simulink model "thrust_allocation"  (R2019a)
settings: Solver=FixedStepAuto  StartTime=0.0  StopTime=10.0  FixedStep=0.1  RelTol=1e-3
undefined symbols (not defined in the file or in its folder): thrusters
settings Model: Creator=den  LastModifiedBy=den

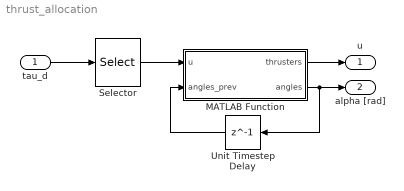
== system thrust_allocation ==
  tau_d : Inport
  MATLAB Function : MATLAB Function  TreatAsAtomicUnit=on
  Selector : Selector  InputPortWidth=6  IndexOptions=Index vector (dialog)  Indices=[1 2 6]  OutputSizes=1
  Unit Timestep Delay : Delay  DelayLength=1  InitialCondition=[thrusters.initangle]
  u : Outport
  alpha [rad] : Outport  Port=2
  wires:
  MATLAB Function/1(thrusters) -> u/1
  Selector/1 -> MATLAB Function/1(u)
  Unit Timestep Delay/1 -> MATLAB Function/2(angles_prev)
  tau_d/1 -> Selector/1
  MATLAB Function/2(angles) -> Unit Timestep Delay/1, alpha [rad]/1

== matlab function thrust_allocation/MATLAB Function ==
  data: u input; thrusters output; angles output; angles_prev input
function [thrusters, angles] = fcn(u, angles_prev)

% thrusters = load('thrusters_sup.mat');
% thrustLimits = [thrusters.thrust];
% throttleLimits = [thrusters.rate];
% turnLimit = [thrusters.rotationspeed];
% 
% % thruster positions
% tp = [thrusters.xposition; thrusters.yposition];

thrustLimits = [125000; 125000; 150000; 320000; 320000];
throttleLimits = [15625; 15625; 18750; 32000; 32000];
turnLimit = [NaN; NaN; 0.209400000000000; 0.209400000000000; 0.209400000000000];

% thruster positions
tp = [[39.3000000000000;35.3000000000000;31.3000000000000;-28.5000000000000;-28.5000000000000] [0;0;0;5;-5]];


mat = [0 0 1 0 1 0 1 0;
       1 1 0 1 0 1 0 1;
       tp(1,1) tp(2,1) 0 tp(3,1) -tp(4,2) tp(4,1) tp(5,2) -tp(5,1)];

% mat_inv = pinv(mat);

W = diag([1, 1, 4, 4, 8, 16, 8, 16]);



mat_inv = (W \ mat') / (mat * (W \ mat'));


y = mat_inv * u;

thrusters = zeros(5,1);
angles = zeros(5,1);

thrusters(1) = y(1);
thrusters(2) = y(2);

thrusters(3) = sqrt(y(3)^2 + y(4)^2);
thrusters(4) = sqrt(y(5)^2 + y(6)^2);
thrusters(5) = sqrt(y(7)^2 + y(8)^2);

angles(1) = 0;
angles(2) = 0;

angles(3) = atan2(y(4), y(3));
angles(4) = atan2(y(6), y(5));
angles(5) = atan2(y(8), y(7));
